simulink model "Appendix_A_CRecovery"  (R2013a)
settings: Solver=ode3  StartTime=0.0  StopTime=10e3/2400  FixedStep=1/480e3  RelTol=1e-3
libraries: dsparch4 x4, commsynccomp2 x3, commfilt2 x3, commsink2 x2, commutil2 x1, commchan3 x1, commrandsrc2 x1, simulink_extras x1, simulink x1
settings Model: Creator=tibbs2010  LastModifiedBy=tibbs2010

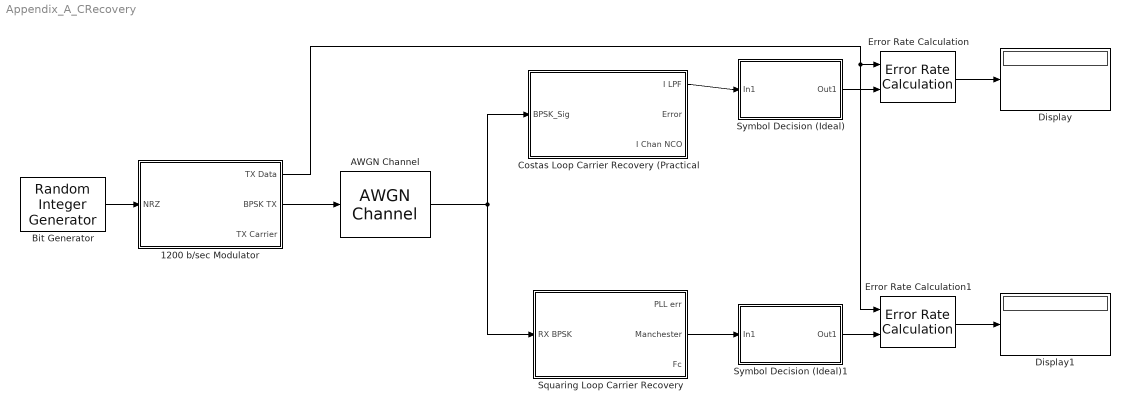
== system Appendix_A_CRecovery ==
  1200 b/sec Modulator : Subsystem
  AWGN Channel : commchan3/AWGN Channel  InputProcessing=Columns as channels (frame based)  seed=randseed  noiseMode="Signal to noise ratio  (Eb/No)"  EbNodB=0  EsNodB=10  SNRdB=10  bitsPerSym=1  Ps=12.5  Tsym=1/2400  variance=1
  Bit Generator : commrandsrc2/Random Integer Generator  mul=2  seed=randseed  Ts=1/2400  frameBased=off  sampPerFrame=1  orient=off  outDataType=double
  Costas Loop Carrier Recovery (Practical : Subsystem
  Display : Display
  Display1 : Display
  Error Rate Calculation : commsink2/Error Rate Calculation  N=3  st_delay=0  cp_mode=Entire frame  subframe=[]  PMode=Port  WsName=ErrorVec  RsMode2=off  stop=off  numErr=100  maxBits=1e6
  Error Rate Calculation1 : commsink2/Error Rate Calculation  N=3  st_delay=0  cp_mode=Entire frame  subframe=[]  PMode=Port  WsName=ErrorVec  RsMode2=off  stop=off  numErr=100  maxBits=1e6
  Squaring Loop Carrier Recovery : Subsystem
  Symbol Decision (Ideal) : Subsystem
  Symbol Decision (Ideal)1 : Subsystem
  wires:
  Bit Generator/1 -> 1200 b/sec Modulator/1(NRZ)
  1200 b/sec Modulator/2(BPSK TX) -> AWGN Channel/1
  AWGN Channel/1 -> Costas Loop Carrier Recovery (Practical/1(BPSK_Sig), Squaring Loop Carrier Recovery/1(RX BPSK)
  Costas Loop Carrier Recovery (Practical/1(I LPF) -> Symbol Decision (Ideal)/1(In1)
  Squaring Loop Carrier Recovery/2(Manchester) -> Symbol Decision (Ideal)1/1(In1)
  Symbol Decision (Ideal)/1(Out1) -> Error Rate Calculation/2
  Error Rate Calculation/1 -> Display/1
  Symbol Decision (Ideal)1/1(Out1) -> Error Rate Calculation1/2
  Error Rate Calculation1/1 -> Display1/1
  1200 b/sec Modulator/1(TX Data) -> Error Rate Calculation1/1, Error Rate Calculation/1

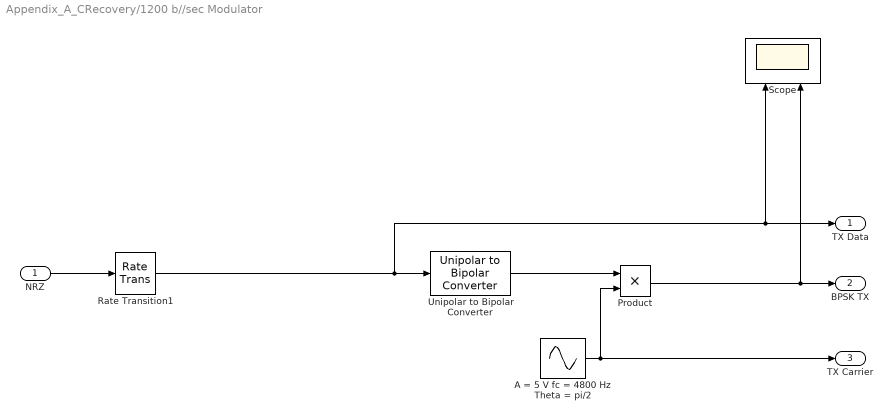
== system Appendix_A_CRecovery/1200 b//sec Modulator ==
  NRZ : Inport
  A = 5 V fc = 4800 Hz Theta = pi/2 : Sin  Amplitude=5  Frequency=2*pi*4800  Phase=pi/2  SampleTime=1/480e3
  Product : Product
  Rate Transition1 : RateTransition  OutPortSampleTime=1/480e3
  Scope : Scope  NumInputPorts=2
      settings: TimeRange=0.06  YMin=-0.5~-0.5  YMax=1.5~1.5  SaveName=ScopeData2
  Unipolar to Bipolar Converter : commutil2/Unipolar to Bipolar Converter  M=2  polarity=Positive  dataType=Inherit via internal rule
  TX Data : Outport
  BPSK TX : Outport  Port=2
  TX Carrier : Outport  Port=3
  wires:
  Rate Transition1/1 -> TX Data/1, Scope/1, Unipolar to Bipolar Converter/1
  Unipolar to Bipolar Converter/1 -> Product/1
  A = 5 V fc = 4800 Hz Theta = pi/2/1 -> TX Carrier/1, Product/2
  NRZ/1 -> Rate Transition1/1
  Product/1 -> Scope/2, BPSK TX/1

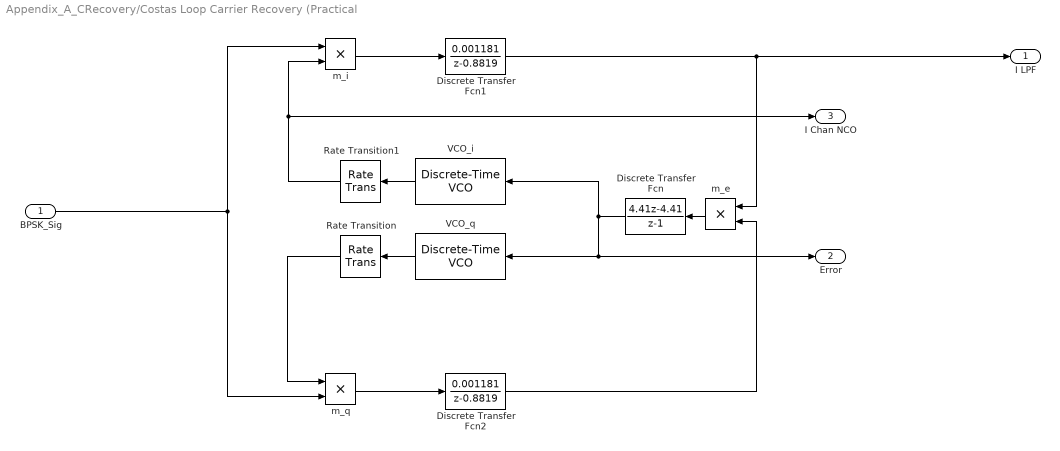
== system Appendix_A_CRecovery/Costas Loop Carrier Recovery (Practical ==
  BPSK_Sig : Inport
  Discrete Transfer Fcn : DiscreteTransferFcn  Numerator=[4.41 -4.41]  Denominator=[1 -1]  SampleTime=1/480e3
  Discrete Transfer Fcn1 : DiscreteTransferFcn  Numerator=[0.001181]  Denominator=[1 -0.8819]  SampleTime=1/480e3
  Discrete Transfer Fcn2 : DiscreteTransferFcn  Numerator=[0.001181]  Denominator=[1 -0.8819]  SampleTime=1/480e3
  Rate Transition : RateTransition  OutPortSampleTime=1/480e3
  Rate Transition1 : RateTransition  OutPortSampleTime=1/480e3
  VCO_i : commsynccomp2/Discrete-Time VCO  Ac=5  Fc=4800  Kc=100  Ph=0  ts=1/480e3
  VCO_q : commsynccomp2/Discrete-Time VCO  Ac=5  Fc=4800  Kc=100  Ph=pi/2  ts=1/480e3
  m_e : Product  SampleTime=1/480e3
  m_i : Product  SampleTime=1/480e3
  m_q : Product  SampleTime=1/480e3
  I LPF : Outport
  Error : Outport  Port=2
  I Chan NCO : Outport  Port=3
  wires:
  VCO_i/1 -> Rate Transition1/1
  VCO_q/1 -> Rate Transition/1
  Rate Transition/1 -> m_q/1
  Rate Transition1/1 -> m_i/2, I Chan NCO/1
  m_q/1 -> Discrete Transfer Fcn2/1
  m_i/1 -> Discrete Transfer Fcn1/1
  BPSK_Sig/1 -> m_i/1, m_q/2
  m_e/1 -> Discrete Transfer Fcn/1
  Discrete Transfer Fcn2/1 -> m_e/2
  Discrete Transfer Fcn/1 -> VCO_i/1, Error/1, VCO_q/1
  Discrete Transfer Fcn1/1 -> I LPF/1, m_e/1

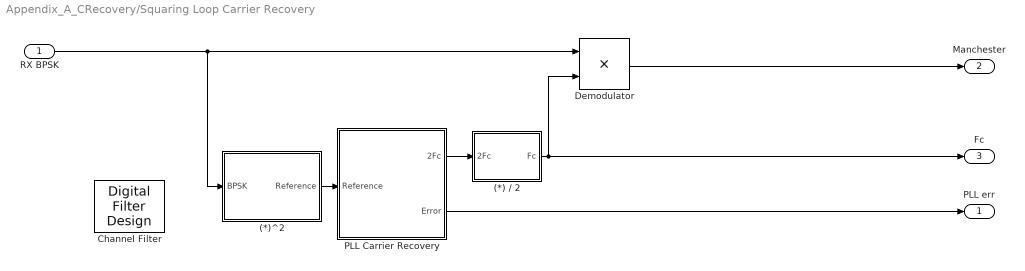
== system Appendix_A_CRecovery/Squaring Loop Carrier Recovery ==
  RX BPSK : Inport
  (*) / 2 : Subsystem
  (*)^2 : Subsystem
  Channel Filter : dsparch4/Digital Filter Design  mwdsp_browser_bugfix_var=off
  Demodulator : Product
  PLL Carrier Recovery : Subsystem
  PLL err : Outport
  Manchester : Outport  Port=2
  Fc : Outport  Port=3
  wires:
  PLL Carrier Recovery/1(2Fc) -> (*) / 2/1(2Fc)
  (*) / 2/1(Fc) -> Demodulator/2, Fc/1
  (*)^2/1(Reference) -> PLL Carrier Recovery/1(Reference)
  Demodulator/1 -> Manchester/1
  RX BPSK/1 -> Demodulator/1, (*)^2/1(BPSK)
  PLL Carrier Recovery/2(Error) -> PLL err/1

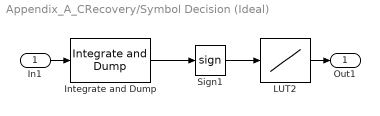
== system Appendix_A_CRecovery/Symbol Decision (Ideal) ==
  In1 : Inport
  Integrate and Dump : commfilt2/Integrate and Dump  obssamples=200  offsetsamples=0  nodump=off  roundingMode=Floor  overflowMode=off
  LUT2 : Lookup_n-D  NumberOfTableDimensions=1  BreakpointsForDimension1=[-1 0 1]  Table=[0 0 1]  RndMeth=Simplest  InputSameDT=on
  Sign1 : Signum
  Out1 : Outport
  wires:
  LUT2/1 -> Out1/1
  In1/1 -> Integrate and Dump/1
  Integrate and Dump/1 -> Sign1/1
  Sign1/1 -> LUT2/1

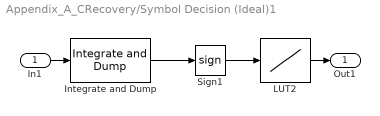
== system Appendix_A_CRecovery/Symbol Decision (Ideal)1 ==
  In1 : Inport
  Integrate and Dump : commfilt2/Integrate and Dump  obssamples=200  offsetsamples=0  nodump=off  roundingMode=Floor  overflowMode=off
  LUT2 : Lookup_n-D  NumberOfTableDimensions=1  BreakpointsForDimension1=[-1 0 1]  Table=[0 0 1]  RndMeth=Simplest  InputSameDT=on
  Sign1 : Signum
  Out1 : Outport
  wires:
  LUT2/1 -> Out1/1
  In1/1 -> Integrate and Dump/1
  Integrate and Dump/1 -> Sign1/1
  Sign1/1 -> LUT2/1

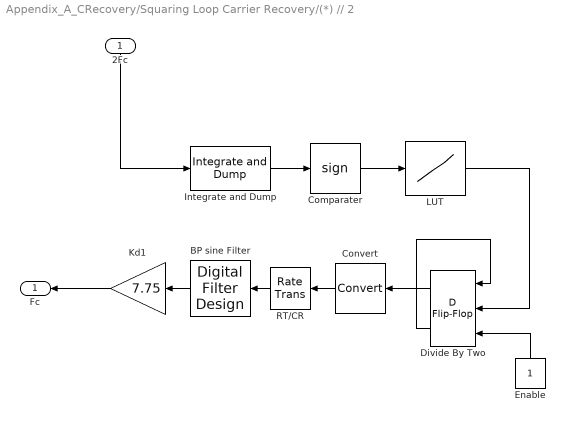
== system Appendix_A_CRecovery/Squaring Loop Carrier Recovery/(*) // 2 ==
  2Fc : Inport
  BP sine Filter : dsparch4/Digital Filter Design  mwdsp_browser_bugfix_var=off
  Comparater : Signum
  Convert : DataTypeConversion
  Divide By Two : simulink_extras/Flip Flops/D Flip-Flop
  Enable : Constant
  Integrate and Dump : commfilt2/Integrate and Dump  obssamples=25  offsetsamples=0  nodump=off  roundingMode=Floor  overflowMode=off
  Kd1 : Gain  Gain=7.75
  LUT : Lookup_n-D  NumberOfTableDimensions=1  BreakpointsForDimension1=[-1 0 1]  Table=[0 0 1]  RndMeth=Simplest  InputSameDT=on
  RT/CR : RateTransition  OutPortSampleTime=1/480e3
  Fc : Outport
  wires:
  Kd1/1 -> Fc/1
  Convert/1 -> RT/CR/1
  RT/CR/1 -> BP sine Filter/1
  Comparater/1 -> LUT/1
  Enable/1 -> Divide By Two/3
  Integrate and Dump/1 -> Comparater/1
  Divide By Two/1 -> Convert/1
  BP sine Filter/1 -> Kd1/1
  LUT/1 -> Divide By Two/2
  Divide By Two/2 -> Divide By Two/1
  2Fc/1 -> Integrate and Dump/1

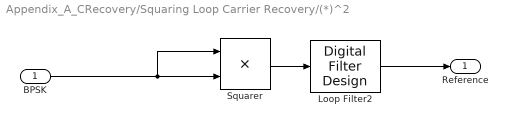
== system Appendix_A_CRecovery/Squaring Loop Carrier Recovery/(*)^2 ==
  BPSK : Inport
  Loop Filter2 : dsparch4/Digital Filter Design  mwdsp_browser_bugfix_var=off
  Squarer : Product
  Reference : Outport
  wires:
  BPSK/1 -> Squarer/2, Squarer/1
  Squarer/1 -> Loop Filter2/1
  Loop Filter2/1 -> Reference/1

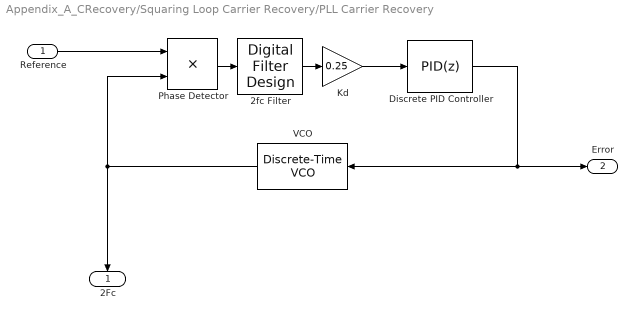
== system Appendix_A_CRecovery/Squaring Loop Carrier Recovery/PLL Carrier Recovery ==
  Reference : Inport
  2fc Filter : dsparch4/Digital Filter Design  mwdsp_browser_bugfix_var=off
  Discrete PID Controller : simulink/Continuous/PID Controller  Controller=PID  TimeDomain=Discrete-time  SampleTime=1/480e3  IntegratorMethod=Forward Euler  FilterMethod=Forward Euler  Form=Parallel  P=5  I=10  D=3  N=1  InitialConditionSource=internal  InitialConditionForIntegrator=0  InitialConditionForFilter=0  ExternalReset=none  LimitOutput=off  UpperSaturationLimit=inf  LowerSaturationLimit=-inf  LinearizeAsGain=off  AntiWindupMode=none  Kb=1  TrackingMode=off  Kt=1  PParamMin=[]  PParamMax=[]  IParamMin=[]  IParamMax=[]  DParamMin=[]  DParamMax=[]  NParamMin=[]  NParamMax=[]  KbParamMin=[]  KbParamMax=[]  KtParamMin=[]  KtParamMax=[]  POutMin=[]  POutMax=[]  IOutMin=[]  IOutMax=[]  DOutMin=[]  DOutMax=[]  NOutMin=[]  NOutMax=[]  KbOutMin=[]  KbOutMax=[]  KtOutMin=[]  KtOutMax=[]  IntegratorOutMin=[]  IntegratorOutMax=[]  FilterOutMin=[]  FilterOutMax=[]  SumOutMin=[]  SumOutMax=[]  SumI1OutMin=[]  SumI1OutMax=[]  SumI2OutMin=[]  SumI2OutMax=[]  SumI3OutMin=[]  SumI3OutMax=[]  SumDOutMin=[]  SumDOutMax=[]  SaturationOutMin=[]  SaturationOutMax=[]  IntegratorContinuousStateAttributes=''  IntegratorStateMustResolveToSignalObject=off  IntegratorRTWStateStorageClass=Auto  FilterContinuousStateAttributes=''  FilterStateMustResolveToSignalObject=off  FilterRTWStateStorageClass=Auto
  Kd : Gain  Gain=0.25
  Phase Detector : Product
  VCO : commsynccomp2/Discrete-Time VCO  Ac=5  Fc=9600  Kc=1  Ph=pi  ts=1/480e3
  2Fc : Outport
  Error : Outport  Port=2
  wires:
  Reference/1 -> Phase Detector/1
  2fc Filter/1 -> Kd/1
  Discrete PID Controller/1 -> Error/1, VCO/1
  Phase Detector/1 -> 2fc Filter/1
  VCO/1 -> Phase Detector/2, 2Fc/1
  Kd/1 -> Discrete PID Controller/1
